simulink model "atsState"  (Simulink 8.0)
settings: Solver=ode45  StartTime=0.0  StopTime=120  FixedStep=0.1  RelTol=1e-3
libraries: Solver_SF x1, simulink x1
settings Model: Creator=think  LastModifiedBy=think
settings SolverCC: AutoInsertRateTranBlk=on
settings OptimizationCC: ExpressionDepthLimit=128
settings DebuggingCC: UnderspecifiedInitializationDetection=Simplified  MergeDetectMultiDrivingBlocksExec=error  SolverPrmCheckMsg=none  FrameProcessingCompatibilityMsg=error  StateNameClashWarn=none
settings HardwareCC: ProdHWDeviceType=Generic->Unspecified (assume 32-bit Generic)
settings ModelReferenceCC: PropagateSignalLabelsOutOfModel=on
settings CodeAppCC: CustomSymbolStrType=$N$R$M_T  InternalIdentifier=Shortened
settings GRTTargetCC: CodeReplacementLibrary=None  CPPClassGenCompliant=on
settings ConfigurationSet: Description=SimMechanics 2G

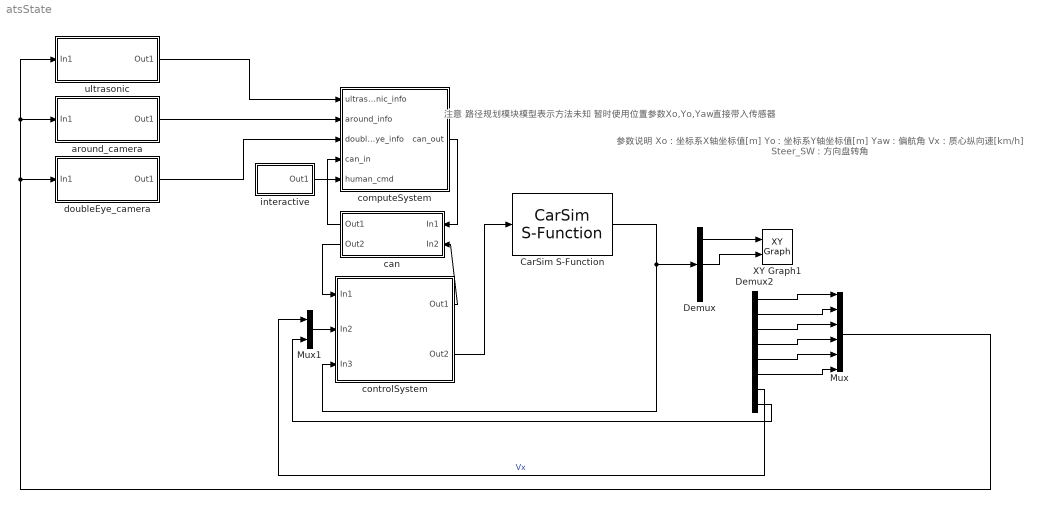
== system atsState ==
  note: 注意
      | 路径规划模块模型表示方法未知
      | 暂时使用位置参数Xo,Yo,Yaw直接带入传感器
  note: 参数说明
      | Xo：坐标系X轴坐标值[m]
      | Yo：坐标系Y轴坐标值[m]
      | Yaw：偏航角
      | Vx：质心纵向速[km/h]
      | Steer_SW：方向盘转角
  CarSim S-Function : Solver_SF/CarSim S-Function  Priority=1  VehicleCode=i_i  SIMFILE=simfile
  Demux : Demux  Outputs=3
  Demux2 : Demux  Outputs=8
  Mux : Mux  Inputs=6
  Mux1 : Mux  Inputs=2
  XY Graph1 : simulink/Sinks/XY Graph  xmin=-50  xmax=50  ymin=-50  ymax=50  st=-1
  around_camera : Subsystem
  can : Subsystem
  computeSystem : Subsystem
  controlSystem : Subsystem
  doubleEye_camera : Subsystem
  interactive : Subsystem
  ultrasonic : Subsystem
  wires:
  Mux/1 -> ultrasonic/1(In1), around_camera/1(In1), doubleEye_camera/1(In1)
  computeSystem/1(can_out) -> can/1(In1)
  can/1(Out1) -> computeSystem/4(can_in)
  can/2(Out2) -> controlSystem/1(In1)
  ultrasonic/1(Out1) -> computeSystem/1(ultrasonic_info)
  around_camera/1(Out1) -> computeSystem/2(around_info)
  doubleEye_camera/1(Out1) -> computeSystem/3(doubleEye_info)
  controlSystem/2(Out2) -> CarSim S-Function/1
  CarSim S-Function/1 -> controlSystem/3(In3), Demux/1
  Demux2/8 -> Mux1/2
  Demux2/6 -> Mux/6
  controlSystem/1(Out1) -> can/2(In2)
  Demux2/5 -> Mux/5
  Demux2/4 -> Mux/4
  Mux1/1 -> controlSystem/2(In2)
  Demux2/3 -> Mux/3
  Demux2/2 -> Mux/2
  Demux2/1 -> Mux/1
  Demux2/7 -> Mux1/1  "Vx"
  interactive/1(Out1) -> computeSystem/5(human_cmd)
  Demux/1 -> XY Graph1/1
  Demux/2 -> XY Graph1/2

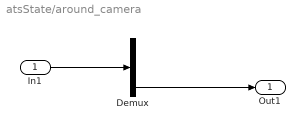
== system atsState/around_camera ==
  In1 : Inport
  Demux : Demux  Outputs=3
  Out1 : Outport
  wires:
  In1/1 -> Demux/1
  Demux/3 -> Out1/1

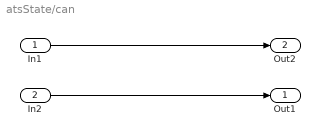
== system atsState/can ==
  In1 : Inport
  In2 : Inport  Port=2
  Out1 : Outport
  Out2 : Outport  Port=2
  wires:
  In1/1 -> Out2/1
  In2/1 -> Out1/1

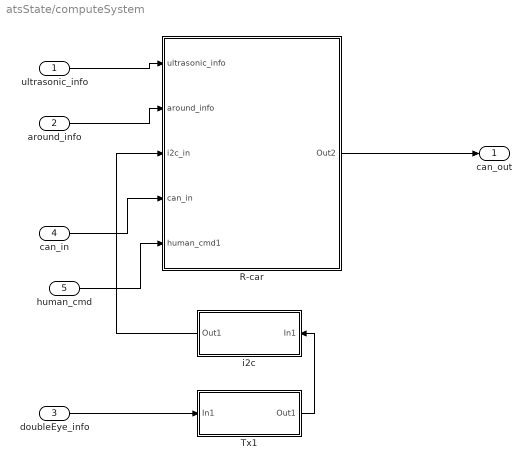
== system atsState/computeSystem ==
  ultrasonic_info : Inport
  around_info : Inport  Port=2
  doubleEye_info : Inport  Port=3
  can_in : Inport  Port=4
  human_cmd : Inport  Port=5
  R-car : Subsystem
  Tx1 : Subsystem
  i2c : Subsystem
  can_out : Outport
  wires:
  ultrasonic_info/1 -> R-car/1(ultrasonic_info)
  doubleEye_info/1 -> Tx1/1(In1)
  around_info/1 -> R-car/2(around_info)
  Tx1/1(Out1) -> i2c/1(In1)
  i2c/1(Out1) -> R-car/3(i2c_in)
  R-car/1(Out2) -> can_out/1
  can_in/1 -> R-car/4(can_in)
  human_cmd/1 -> R-car/5(human_cmd1)

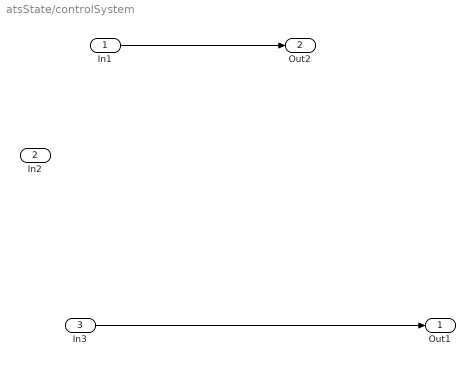
== system atsState/controlSystem ==
  In1 : Inport
  In2 : Inport  Port=2
  In3 : Inport  Port=3
  Out1 : Outport
  Out2 : Outport  Port=2
  wires:
  In3/1 -> Out1/1
  In1/1 -> Out2/1

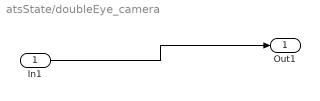
== system atsState/doubleEye_camera ==
  In1 : Inport
  Out1 : Outport
  wires:
  In1/1 -> Out1/1

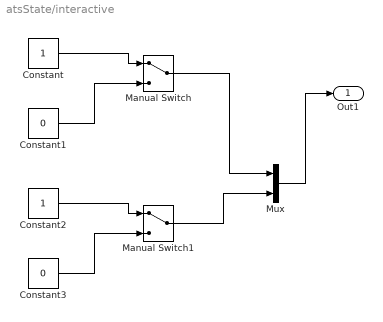
== system atsState/interactive ==
  Constant : Constant
  Constant1 : Constant  Value=0
  Constant2 : Constant
  Constant3 : Constant  Value=0
  Manual Switch : ManualSwitch
  Manual Switch1 : ManualSwitch
  Mux : Mux  Inputs=2
  Out1 : Outport
  wires:
  Constant1/1 -> Manual Switch/2
  Constant/1 -> Manual Switch/1
  Manual Switch/1 -> Mux/1
  Constant3/1 -> Manual Switch1/2
  Constant2/1 -> Manual Switch1/1
  Manual Switch1/1 -> Mux/2
  Mux/1 -> Out1/1

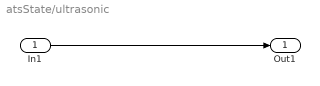
== system atsState/ultrasonic ==
  In1 : Inport
  Out1 : Outport
  wires:
  In1/1 -> Out1/1

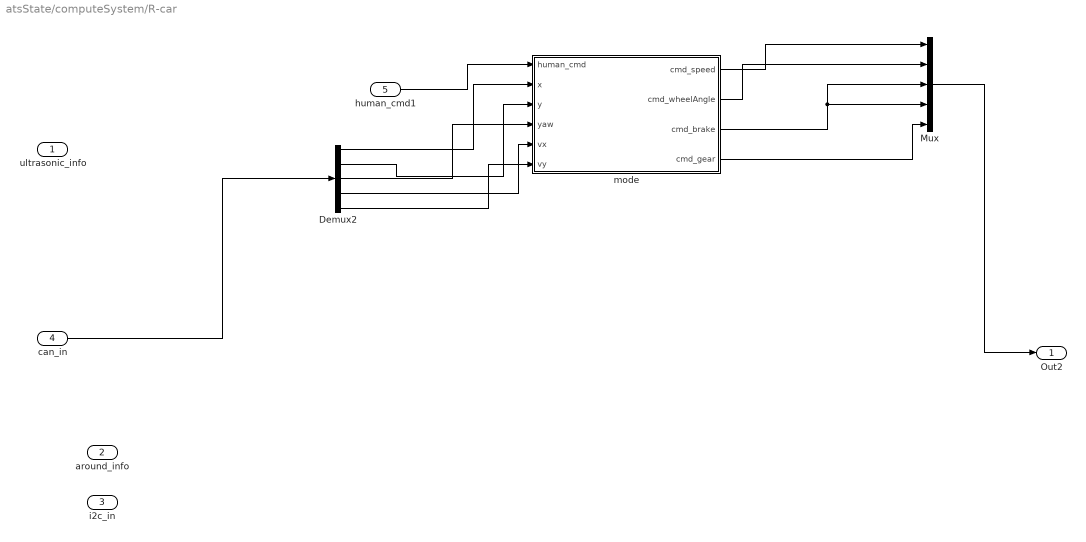
== system atsState/computeSystem/R-car ==
  ultrasonic_info : Inport
  around_info : Inport  Port=2
  i2c_in : Inport  Port=3
  can_in : Inport  Port=4
  human_cmd1 : Inport  Port=5
  Demux2 : Demux  Outputs=5
  Mux : Mux  Inputs=5
  mode : Stateflow chart  TreatAsAtomicUnit=on
  Out2 : Outport
  wires:
  human_cmd1/1 -> mode/1(human_cmd)
  mode/1(cmd_speed) -> Mux/1
  mode/2(cmd_wheelAngle) -> Mux/2
  mode/3(cmd_brake) -> Mux/4, Mux/3
  mode/4(cmd_gear) -> Mux/5
  Demux2/1 -> mode/2(x)
  Demux2/2 -> mode/3(y)
  Demux2/3 -> mode/4(yaw)
  Mux/1 -> Out2/1
  can_in/1 -> Demux2/1
  Demux2/4 -> mode/5(vx)
  Demux2/5 -> mode/6(vy)

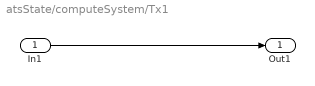
== system atsState/computeSystem/Tx1 ==
  In1 : Inport
  Out1 : Outport
  wires:
  In1/1 -> Out1/1

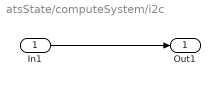
== system atsState/computeSystem/i2c ==
  In1 : Inport
  Out1 : Outport
  wires:
  In1/1 -> Out1/1

== stateflow chart computeSystem/R-car/mode ==
  state automative_parking
    state routing
      state going_stright
        state finding_port
        (default) -> finding_port
        finding_port -> finding_port [order 2] : [x<10&&y<10&&value==0]
            | {out(50,0,0,4);}
      (default) -> going_stright
    state parkping
      state holding
      state executing
        (junction 42) -> (junction 41) : {out(-10,cmd_wheelAngle,0,0);}
        (junction 43) -> (junction 42) [order 1] : [yaw>=90]
            | {cmd_wheelAngle=0;
            | done=1;}
        (junction 43) -> (junction 42) [order 2] : [yaw<90]
            | {cmd_wheelAngle=-540;}
        (default) -> (junction 43)
      state adjusting
        (default) -> (junction 48) : {out(-10,0,0,0);
            | done=done+1;}
      (default) -> holding
      holding -> (junction 34) [order 2] : [done==0]
      adjusting -> holding : [y<-5]
      (junction 34) -> executing
      executing -> holding
      holding -> adjusting [order 1] : [done==1||done==2]
    state stopping
    state complete
    (default) -> routing
    finding_port -> stopping [order 1] : [x>=10||y>=10]
        | {value=1;}
    stopping -> (junction 16) [order 2] : [(vx<=0.1&&vy<=0.1)&&(vx>=-0.1&&vy>=-0.1)]
    (junction 16) -> stopping [order 3]
    (junction 16) -> complete [order 1] : [done==3]
    (junction 16) -> parkping [order 2] : [done<=2]
        | {done=done+1;}
    holding -> stopping [order 3] : [done==3]
    stopping -> stopping [order 1] : [(vx>0.1||vy>0.1)||(vx<-0.1||vy<-0.1)||cmd_speed!=0]
        | {out(0,0,4,0);}
  state dead
  state out(s,a,b,g) [function]
    (default) -> (junction 30) : {cmd_speed=s;
        | cmd_wheelAngle=a;
        | cmd_gear=g;
        | cmd_brake=b;}
  note: 车的状态？模式？
      | 输出：
      |
      | 档位
      | 刹车指令
      | 方向盘角度
      | 速度
      |
      | 未知：
      | simulink function使用
      | 参数向外传递
      |
      | 计划：
      | 先内部排除语法错误
      | 模拟运行无问题再出去
  (default) -> dead
  dead -> automative_parking : [human_cmd[0]==1&&done!=3]
  complete -> dead
  data: s function_input double; a function_input double; b function_input double; g function_input double; cmd_speed output int32; cmd_wheelAngle output int32; cmd_brake output int32; human_cmd input double; x input double; cmd_gear output int32; y input double; yaw input double; value local double =0; done local double =-1; vx input double; vy input double
  events: finish local RISING_EDGE_EVENT; stopped local RISING_EDGE_EVENT
